simulink model "embedded_with_end"  (Simulink 7.6)
settings: Solver=FixedStepDiscrete  StartTime=0.0  StopTime=10.0  FixedStep=1  RelTol=1e-3
settings Model: Creator=Harmon S. Nine  LastModifiedBy=c2wt
settings DebuggingCC: StrictBusMsg=Warning
settings SFSimCC: SimParseCustomCode=off

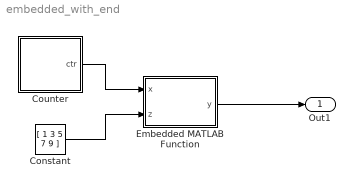
== system embedded_with_end ==
  Constant : Constant  Value=[ 1 3 5 7 9 ]  VectorParams1D=off
  Counter : Stateflow chart  TreatAsAtomicUnit=on
  Embedded MATLAB Function : Stateflow chart  TreatAsAtomicUnit=on
  Out1 : Outport
  wires:
  Embedded MATLAB Function/1(y) -> Out1/1
  Counter/1(ctr) -> Embedded MATLAB Function/1(x)
  Constant/1 -> Embedded MATLAB Function/2(z)

== stateflow chart Counter ==
  state s1
  (default) -> s1
  s1 -> s1 [order 1] : [ctr < 4] / ctr = ctr+1;
  s1 -> s1 [order 2] : [ctr >= 4] / ctr = 0;
  data: ctr output double =1

== matlab function Embedded MATLAB Function ==
  data: y output double; x input double; z input double
function y = fcn(x,z)
%#eml

y = z( end - x );
